simulink model "PF_core_control"  (R2023b)
settings: configuration reference "slow_tsk_conf" (kept outside this file)
undefined symbols (not defined in the file): slow_tsk_st
libraries: eeGeneralControl x1
settings Model: DataDictionary=fmuGenerationDictionay.sldd  ModifiedByFormat=Third Equation Ltd  Creator=Third Equation Ltd  LastModifiedBy=Third Equation Ltd
settings ConfigSetRef: SourceName=slow_tsk_conf

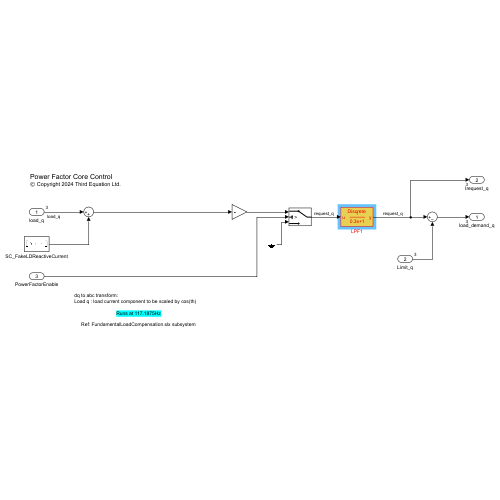
[thumbnail: Simulink's stored preview of the top-level diagram]
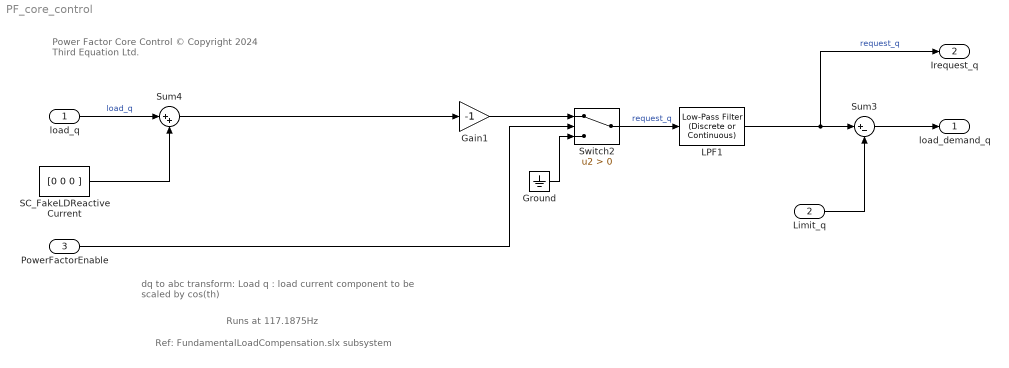
== system PF_core_control ==
  note: dq to abc transform:
      | Load q : load current component to be scaled by cos(th)
  note: Power Factor Core Control
      | © Copyright 2024 Third Equation Ltd.
  note: Runs at 117.1875Hz
  note: Ref: FundamentalLoadCompensation.slx subsystem
  load_q : Inport  OutDataTypeStr=single  PortDimensions=3
  Limit_q : Inport  Port=2  OutDataTypeStr=single  PortDimensions=3
  PowerFactorEnable : Inport  Port=3  OutDataTypeStr=boolean  PortDimensions=1
  Gain1 : Gain  Gain=-1
  Ground : Ground
  LPF1 : eeGeneralControl/Low-Pass Filter (Discrete or Continuous)  K=1  T=0.3  B=inf  A=-inf  init_option=Inherited from block input  x0=0  Ts=slow_tsk_st
  SC_FakeLDReactiveCurrent : Constant  Value=[0 0 0 ]  OutDataTypeStr=single
  Sum3 : Sum  Inputs=|+-
  Sum4 : Sum  Inputs=|++
  Switch2 : Switch  Criteria=u2 > Threshold  SaturateOnIntegerOverflow=off  InputSameDT=off
  load_demand_q : Outport  OutDataTypeStr=single  PortDimensions=3
  Irequest_q : Outport  Port=2  OutDataTypeStr=single  PortDimensions=3
  wires:
  Ground/1 -> Switch2/3
  Gain1/1 -> Switch2/1
  Switch2/1 -> LPF1/1  "request_q"
  SC_FakeLDReactiveCurrent/1 -> Sum4/2
  load_q/1 -> Sum4/1  "load_q"
  PowerFactorEnable/1 -> Switch2/2
  LPF1/1 -> Sum3/1, Irequest_q/1  "request_q"
  Sum4/1 -> Gain1/1
  Limit_q/1 -> Sum3/2
  Sum3/1 -> load_demand_q/1
